simulink model "ADRC1"  (Simulink 8.8)
settings: Solver=ode3  StartTime=0.0  StopTime=10  FixedStep=0.01  RelTol=1e-3  EnableMultiTasking=on
libraries: simulink x1
settings Model: Creator=lenovo  LastModifiedBy=LZ
settings OptimizationCC: InitFltsAndDblsToZero=on
settings DebuggingCC: SaveWithParameterizedLinksMsg=none  SignalResolutionControl=TryResolveAllWithWarning  SolverPrmCheckMsg=warning  MultiTaskDSMMsg=warning  MultiTaskCondExecSysMsg=none  StateNameClashWarn=none
settings GRTTargetCC: TargetFcnLib=ansi_tfl_tmw.mat  GeneratePreprocessorConditionals=Use local settings

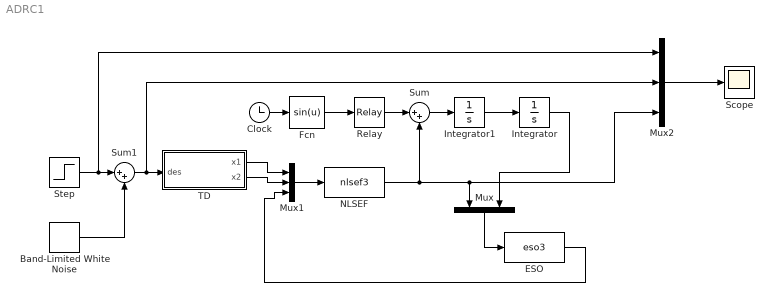
== system ADRC1 ==
  Band-Limited White Noise : simulink/Sources/Band-Limited White Noise  Cov=0.0001  Ts=0.01  seed=[23341]
  Clock : Clock
  ESO : S-Function  FunctionName=eso3  Parameters=d,bet,b  SFunctionDeploymentMode=off  EnableBusSupport=off  mask{bet=[100;65;80], d=0, b=1}
  Fcn : Fcn  Expr=sin(u)
  Integrator : Integrator
  Integrator1 : Integrator
  Mux : Mux  Inputs=2
  Mux1 : Mux  Inputs=3
  Mux2 : Mux  Inputs=3
  NLSEF : S-Function  FunctionName=nlsef3  Parameters=aa,bet1,b,d  SFunctionDeploymentMode=off  EnableBusSupport=off  mask{bet1=[100;10], aa=[0.75;1.25], b=1, d=0}
  Relay : Relay
  Scope : Scope
  Step : Step  Time=2  SampleTime=0
  Sum : Sum  Inputs=|++  SaturateOnIntegerOverflow=on  InputSameDT=on  OutDataTypeStr=Inherit: Same as first input
  Sum1 : Sum  Inputs=|++
  TD : Subsystem
  wires:
  Clock/1 -> Fcn/1
  Sum/1 -> Integrator1/1
  Integrator1/1 -> Integrator/1
  Integrator/1 -> Mux/2
  Fcn/1 -> Relay/1
  Relay/1 -> Sum/1
  Sum1/1 -> TD/1(des), Mux2/2
  NLSEF/1 -> Mux2/3, Mux/1, Sum/2
  Mux/1 -> ESO/1
  TD/1(x1) -> Mux1/1
  ESO/1 -> Mux1/3
  Mux1/1 -> NLSEF/1
  Mux2/1 -> Scope/1
  Step/1 -> Mux2/1, Sum1/1
  Band-Limited White Noise/1 -> Sum1/2
  TD/2(x2) -> Mux1/2

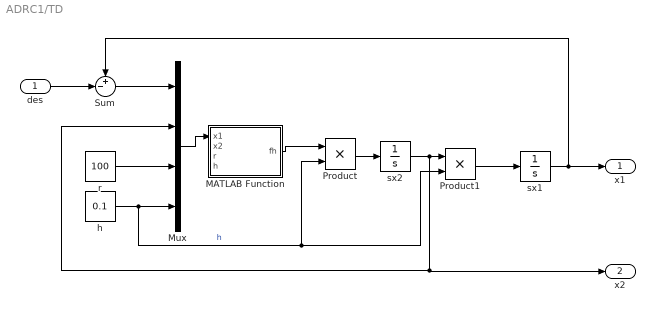
== system ADRC1/TD ==
  des : Inport
  MATLAB Function : MATLAB Function  TreatAsAtomicUnit=on
  Mux : Mux
  Product : Product
  Product1 : Product
  Sum : Sum  Inputs=+-|
  h : Constant  Value=0.1
  r : Constant  Value=100
  sx1 : Integrator
  sx2 : Integrator
  x1 : Outport
  x2 : Outport  Port=2
  wires:
  sx2/1 -> x2/1, Mux/2, Product1/1
  h/1 -> Product/2, Product1/2, Mux/4  "h"
  Product/1 -> sx2/1
  MATLAB Function/1(fh) -> Product/1
  sx1/1 -> x1/1, Sum/1
  r/1 -> Mux/3
  Product1/1 -> sx1/1
  Mux/1 -> MATLAB Function/1(x1)
  Sum/1 -> Mux/1
  des/1 -> Sum/2

== matlab function TD/MATLAB Function ==
  data: x1 input double; fh output double; x2 input double; r input double; h input double
function  fh = fhan(x1, x2, r, h)
     d = r*h;
     d0 = h*d;
     y = x1 + h*x2;
     a0 = sqrt(d*d +8*r*abs(y));
     
     if abs(y)>d0
         a = x2 + (a0 - d)*sign(y)/2;
     else 
         a = x2 + y/h;
     end
     
     if abs(a)>d
         fh = -r*sign(a);
     else
         fh = -r*a/d;
     end
end
